simulink model "quaternionPropagate"  (R2023b)
settings: Solver=VariableStepAuto  StartTime=0.0  StopTime=Tfinal  RelTol=1e-3
values from neighbouring files (symbols this model uses):
  q0 = [0 0 1 0].'    [quatUnitTest.m]
settings Model: Creator=stanforduser  LastModifiedBy=kristopherriordan
settings DataIOCC: OutputSaveName=R

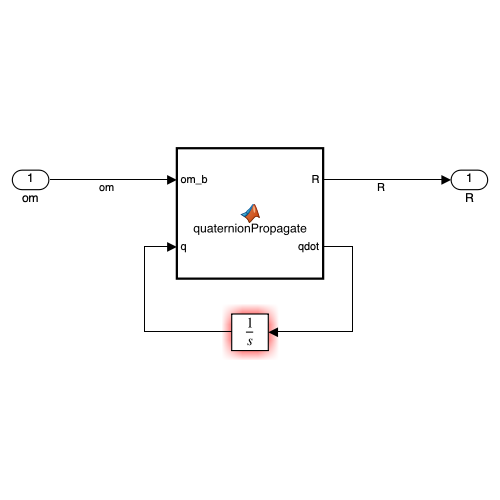
[thumbnail: Simulink's stored preview of the top-level diagram]
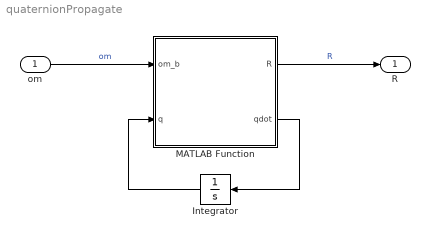
== system quaternionPropagate ==
  om : Inport
  Integrator : Integrator  InitialCondition=q0
  MATLAB Function : MATLAB Function  TreatAsAtomicUnit=on
  R : Outport
  wires:
  om/1 -> MATLAB Function/1(om_b)  "om"
  MATLAB Function/1(R) -> R/1  "R"
  MATLAB Function/2(qdot) -> Integrator/1
  Integrator/1 -> MATLAB Function/2(q)

== matlab function quaternionPropagate/MATLAB Function ==
  data: om_b input size=[3 1]; q input; R output; qdot output
function [R, qdot] = quaternionPropagate(om_b, q)

% udot = zeros(size(u));
q = q./norm(q);
q0 = q(1);
q1 = q(2);
q2 = q(3);
q3 = q(4);
% qvec = q(2:end);

% om1 = om_b(1);
% om2 = om_b(2);
% om3 = om_b(3);

% Om = [0, om3, -om2, om1;
%       -om3, 0, om1, om2;
%       om2, -om1, 0, om3;
%       -om1, -om2, -om3 0];

W_prime = [-q1, q0, q3, -q2;
            -q2, -q3, q0, q1;
            -q3, q2, -q1, q0];

qdot = (1/2)*(W_prime.')*om_b;

% qdot = (1/2).*(Om * q);

% R = (q0^2 - norm(qvec)^2).*eye(3) + 2*qvec*qvec.T - 2*q0

R = [q0^2 + q1^2 - q2^2 - q3^2, 2*q1*q2 + 2*q0 *q3, 2*(q1*q3 - q0*q2);
    2*(q1*q2 - q0*q3), q0^2 - q1^2 + q2^2 - q3^2, 2*(q2*q3 + q0*q1);
    2*(q1*q3 + q0*q2), 2*(q2*q3 - q0*q1), q0^2 - q1^2 - q2^2 + q3^2];
